simulink model "DivideNConquer"  (R2023a)
settings: Solver=VariableStepAuto  StartTime=0  StopTime=6012  MinStep=1e-2  RelTol=1e-3  AbsTol=1e-9
model workspace (MAT data in the model file):
  Cap = 4
  Grade = 0
  QHbatt = 70
  QLbatt = 40
  Trqmax = 400
  Vref = 650
values from neighbouring files (symbols this model uses):
  s = (id-1)*n_sim + 1    [LHSdesign.m]
undefined symbols (not defined in the file or in its folder): Qbatt, Vbatt
libraries: fl_lib x29, nesl_utility x15, sdl_lib x9, ee_lib x7, batteryecm_lib x1, autolibshared x1, slpidlib x1
(part 2 of 2)

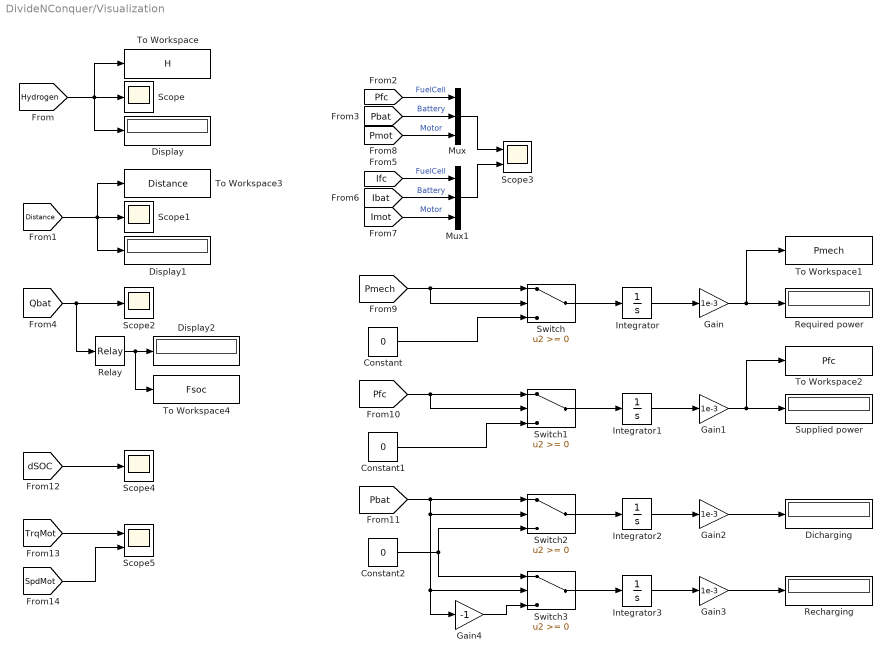
== system DivideNConquer/Visualization ==
  Constant : Constant  Value=0
  Constant1 : Constant  Value=0
  Constant2 : Constant  Value=0
  Dicharging : Display
  Display : Display
  Display1 : Display
  Display2 : Display
  Gain{,1..3} (4 alike) : Gain  Gain=1e-3
  Gain4 : Gain  Gain=-1
  Integrator{,1..3} (4 alike) : Integrator
  Mux : Mux  Inputs=3
  Mux1 : Mux  Inputs=3
  Recharging : Display
  Relay : Relay  OnSwitchValue=100  OffSwitchValue=0
  Required power : Display
  Scope{,1..2,4} (4 alike) : Scope
  Scope3 : Scope  NumInputPorts=2
  Scope5 : Scope  NumInputPorts=2
  Supplied power : Display
  Switch{,1..3} (4 alike) : Switch  SaturateOnIntegerOverflow=off  InputSameDT=off
  To Workspace : ToWorkspace  VariableName=H  SampleTime=-1
      settings: MaxDataPoints=1  Decimation=6  Save2DSignal=2-D array (concatenate along first dimension)
  To Workspace1 : ToWorkspace  VariableName=Pmech  SampleTime=-1
      settings: MaxDataPoints=1  Decimation=6  Save2DSignal=2-D array (concatenate along first dimension)
  To Workspace2 : ToWorkspace  VariableName=Pfc  SampleTime=-1
      settings: MaxDataPoints=1  Decimation=6  Save2DSignal=2-D array (concatenate along first dimension)
  To Workspace3 : ToWorkspace  VariableName=Distance  SampleTime=-1
      settings: MaxDataPoints=1  Decimation=6  Save2DSignal=2-D array (concatenate along first dimension)
  To Workspace4 : ToWorkspace  VariableName=Fsoc  SampleTime=-1
      settings: MaxDataPoints=1  Decimation=6  Save2DSignal=2-D array (concatenate along first dimension)
  wires:
  [Hydrogen] -> To Workspace/1, Display/1, Scope/1
  [Distance] -> To Workspace3/1, Display1/1, Scope1/1
  [Qbat] -> Relay/1, Scope2/1
  Relay/1 -> To Workspace4/1, Display2/1
  [Pmot] -> Mux/3  "Motor"
  Mux1/1 -> Scope3/2
  [Imot] -> Mux1/3  "Motor"
  [Ibat] -> Mux1/2  "Battery"
  [Pfc] -> Mux/1  "FuelCell"
  Mux/1 -> Scope3/1
  [Pbat] -> Mux/2  "Battery"
  [Ifc] -> Mux1/1  "FuelCell"
  Integrator/1 -> Gain/1
  [Pmech] -> Switch/1, Switch/2
  Constant/1 -> Switch/3
  Constant1/1 -> Switch1/3
  Switch1/1 -> Integrator1/1
  Switch/1 -> Integrator/1
  [Pfc] -> Switch1/1, Switch1/2
  Gain/1 -> To Workspace1/1, Required power/1
  Switch3/1 -> Integrator3/1
  Constant2/1 -> Switch3/1, Switch2/3
  [Pbat] -> Switch2/1, Switch2/2, Gain4/1, Switch3/2
  Switch2/1 -> Integrator2/1
  Integrator1/1 -> Gain1/1
  Gain1/1 -> To Workspace2/1, Supplied power/1
  Integrator2/1 -> Gain2/1
  Gain2/1 -> Dicharging/1
  Integrator3/1 -> Gain3/1
  Gain3/1 -> Recharging/1
  Gain4/1 -> Switch3/3
  [dSOC] -> Scope4/1
  [TrqMot] -> Scope5/1
  [SpdMot] -> Scope5/2

== system DivideNConquer/qH2 Control ==
  PS Ramp1 : fl_lib/Physical Signals/Sources/PS Ramp  slope=400/120 lpm/s  start_time=0 s  initial_output=2 lpm
  PS Saturation : fl_lib/Physical Signals/Nonlinear Operators/PS Saturation  upper_limit=300 lpm  lower_limit=2 lpm
  qH2 : PMIOPort  Side=Right
  connections:
  PS Saturation/RConn1 -- qH2/RConn1
  PS Ramp1/RConn1 -- PS Saturation/LConn1
